simulink model "qss_saab93_ideal"  (R2016b)
settings: Solver=VariableStepDiscrete  StartTime=0.0  StopTime=1220  RelTol=1e-3  EnableMultiTasking=on
undefined symbols (not defined in the file or in its folder): eta_ice, g, h, H_u, k_cs, P_CE_idle, P_CE_recup, rho, rho_f
settings Model: Creator=grauers  LastModifiedBy=grauers
settings DataIOCC: LimitDataPoints=on  SaveFormat=Array  SignalLoggingSaveFormat=ModelDataLogs
settings OptimizationCC: InitFltsAndDblsToZero=on  LifeSpan=inf
settings DebuggingCC: SaveWithParameterizedLinksMsg=none  UnderspecifiedInitializationDetection=Classic  MergeDetectMultiDrivingBlocksExec=none  SignalResolutionControl=TryResolveAllWithWarning  SolverPrmCheckMsg=warning  MultiTaskDSMMsg=warning  MultiTaskCondExecSysMsg=none  FcnCallInpInsideContextMsg=warning  SFUnexpectedBacktrackingDiag=warning  SFNoUnconditionalDefaultTransitionDiag=warning  SFExecutionAtInitializationDiag=none
settings HardwareCC: ProdBitPerPointer=32  ProdBitPerSizeT=32  ProdBitPerPtrDiffT=32  ProdLargestAtomicFloat=None  ProdIntDivRoundTo=Undefined  ProdEndianess=Unspecified  ProdWordSize=32  ProdHWDeviceType=32-bit Generic
settings ModelReferenceCC: PropagateSignalLabelsOutOfModel=off
settings GRTTargetCC: TargetFcnLib=ansi_tfl_tmw.mat  TargetLangStandard=C89/C90 (ANSI)  CombineOutputUpdateFcns=off  GRTInterface=on
settings ConfigComp: CovMetricSettings=dw  CovHtmlReporting=on  CovSaveCumulativeToWorkspaceVar=on  CovSaveSingleToWorkspaceVar=on  CovExternalEMLEnable=off

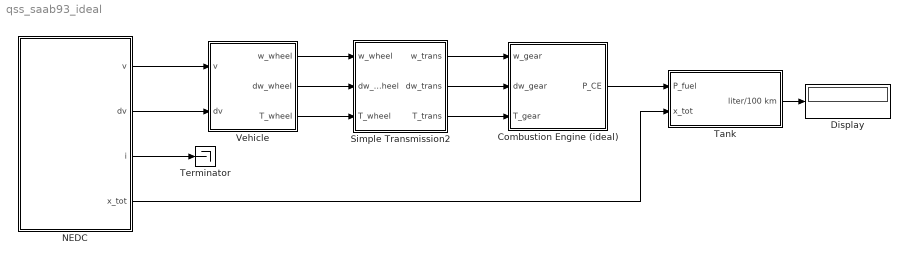
== system qss_saab93_ideal ==
  Combustion Engine (ideal) : Subsystem  Tag=combustion engine  mask(Combustion Engine (ideal)){engine_type=Otto, theta_CE=0.05, P_aux=0, recuperation=No_recuperation, idling=on, idle_power=2600}
      mask prompts: engine_type "Engine type"; theta_CE "Engine inertia [kg*m^2]"; P_aux "Power required by auxiliaries [W]"; recuperation "Recuperation of energy"; idling "Idling power consumption"; idle_power "Idling power consumption [W]"
      mask help:
      | This block simulates the behaviour of a combustion engine. The block is based on an ideal power supply. If engine type ideal is selected then the engine efficiency is 1, else it is 0.4 for otto and 0.5 for diesel.
      |
      | Input:
      | =====
      | 	w_gear		Speed of the fly wheel [rad/s]
      | 	dw_gear	Acceleration of the fly wheel [rad/s^2]
      | 	T_gear		Torque on the fly wheel [Nm]
      |
      | Output:
      | ======
      | 	P_CE		Power produced by the combustion engine [W]
      mask init:
      | init_CE_ideal;
      mask TypeOptions engine_type: Otto | Diesel
      mask TypeOptions recuperation: No_recuperation | Perfect_recuperation
  Display : Display
  NEDC : Subsystem  Tag=cycle  mask(Driving Cycle){cyclename1=NEDC, stepsize=1, autostop=on}
      mask prompts: cyclename1 "Choose a cycle"; stepsize "Step size [s]"; autostop "Enable automatic simulation stop"
      mask help:
      | This block loads the cycle data such as time, speed, acceleration and gear number,  from the specified data file and makes it available on the output of the cycle block.
      |
      | Output:
      | ======
      | 	v	Speed [m/s]
      | 	dv	Acceleration [m/s^2]
      | 	i	Gear number [-]
      | 	x_tot	Total distance [m]
      |
      | Tip:
      | ===
      | Probably you don't need the gear number "i". If so you can terminate
      | it with a "Terminator" out of the "Simulink Library/Connections."
      |
      | Driving cycle:
      | ===
      | Select a driving cycle from the list below or specify your own (place your .mat file in the
      | directory Data/DrivingCycles/UserDefined)
      |
      | ECE_MAN
      | ECE_R15s
      | ECE_R15
      | EUDC
      | EUDC_MAN
      | City
      | City_MAN
      | NEDC
      | NEDC_MANl
      | GOT1
      | GOT2
      | GOT3
      | 10_15_MODE
      | 10_MODE
      | 10_MODE_3
      | 11_MODE
      | 11_MODE_4
      | 15_MODE
      | City_I
      | City_II
      | FTP_75
      | FTP_Highway
      |
      |
      | Step size:
      | ========
      | Default value is 1. Don't change it, unless you are familiar with the programs of the QSS TB.
      |
      | Enable automatic simulation stop:
      | ===========================
      | Stops the simulation automatically at the end of the cycle.
      | Be careful: If you have a component in your model that has to run after the cycle has finished, e.g. a battery to charge, remove the mark!
      mask init:
      | init_driving_cycle1;
      mask Display: plot(T_zplot, V_zplot);
  Simple Transmission2 : Subsystem  Tag=simple transmission  mask(Simple Transmission2){}
      mask help:
      | This block simulates an ideal transmission (no losses).
      |
      | Input:
      | =====
      | 	w_wheel	Speed of the wheel [rad/s]
      | 	dw_wheel	Acceleration of the wheel [rad/s^2]
      | 	T_wheel	Torque on the wheel [Nm]
      |
      | Output:
      | ======
      | 	w_trans		Speed of the fly wheel [rad/s]
      | 	dw_trans	Acceleration of the fly wheel [rad/s^2]
      | 	T_trans		Torque on the fly wheel [Nm]
      mask init:
      | init_transmission;
  Tank : Subsystem  Tag=tank  mask(Tank){fuel=Gasoline, flag_cold_start=off}
      mask prompts: flag_cold_start "Include cold start losses"
      mask help:
      | This block integrates the power (the fuel mass flow) required by the combustion engine or the fuel cell and calculates the energy consumption in liter/100 km.
      |
      | Input:
      | =====
      | 	P_fuel	Power (fuel mass flow) required [W]
      | 	x_tot	Total distance [m]
      |
      | Output:
      | ======
      | 	V	Fuel consumption [liter/100 km]
      mask init:
      | init_tank;
      mask TypeOptions fuel: Gasoline | Diesel | Hydrogen
  Terminator : Terminator
  Vehicle : Subsystem  Tag=vehicle  mask(Vehicle){m_f=1295+80+100, mt2m_f=5, A_f=2, d_wheel=0.62, cw=0.3, mu=0.013}
      mask prompts: m_f "Total mass of the vehicle [kg]"; mt2m_f "Rotating mass [%]"; A_f "Vehicle cross section [m^2]"; d_wheel "Wheel diameter [m]"; cw "Drag coefficient [-]"; mu "Rolling friction coefficient [-]"
      mask help:
      | This block computes the power required from the vehicle.
      |
      | Input:
      | =====
      | 	v		Speed [m/s]
      | 	dv		Acceleration [m/s^2]
      |
      | Output:
      | ======
      | 	w_wheel	Speed of the wheel [rad/s]
      | 	dw_wheel	Acceleration of the wheel [rad/s^2]
      | 	T_wheel	Torque on the wheel [Nm]
      mask init:
      | init_vehicle;
  wires:
  Vehicle/1(w_wheel) -> Simple Transmission2/1(w_wheel)
  Vehicle/2(dw_wheel) -> Simple Transmission2/2(dw_wheel)
  Vehicle/3(T_wheel) -> Simple Transmission2/3(T_wheel)
  Simple Transmission2/1(w_trans) -> Combustion Engine (ideal)/1(w_gear)
  Simple Transmission2/2(dw_trans) -> Combustion Engine (ideal)/2(dw_gear)
  Simple Transmission2/3(T_trans) -> Combustion Engine (ideal)/3(T_gear)
  Tank/1(liter/100 km) -> Display/1
  Combustion Engine (ideal)/1(P_CE) -> Tank/1(P_fuel)
  NEDC/4(x_tot) -> Tank/2(x_tot)
  NEDC/1(v) -> Vehicle/1(v)
  NEDC/2(dv) -> Vehicle/2(dv)
  NEDC/3(i) -> Terminator/1

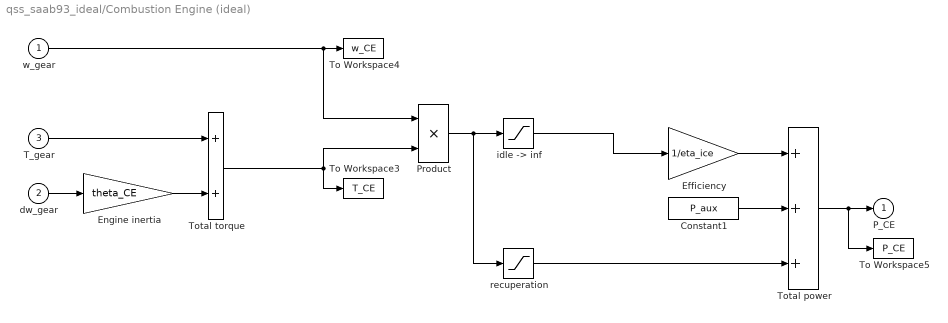
== system qss_saab93_ideal/Combustion Engine (ideal) ==
  w_gear : Inport
  dw_gear : Inport  Port=2
  T_gear : Inport  Port=3
  Constant1 : Constant  Value=P_aux
  Efficiency : Gain  Gain=1/eta_ice  SaturateOnIntegerOverflow=on  OutDataTypeStr=Inherit: Same as input  ParamDataTypeStr=Inherit: Same as input
  Engine inertia : Gain  Gain=theta_CE  SaturateOnIntegerOverflow=on  OutDataTypeStr=Inherit: Same as input  ParamDataTypeStr=Inherit: Same as input
  Product : Product  RndMeth=Zero
  To Workspace3 : ToWorkspace  VariableName=T_CE  SampleTime=-1
  To Workspace4 : ToWorkspace  VariableName=w_CE  SampleTime=-1
  To Workspace5 : ToWorkspace  VariableName=P_CE  SampleTime=-1
  Total power : Sum  Inputs=+++  SaturateOnIntegerOverflow=on  InputSameDT=on  OutDataTypeStr=Inherit: Same as first input
  Total torque : Sum  SaturateOnIntegerOverflow=on  InputSameDT=on  OutDataTypeStr=Inherit: Same as first input
  "idle -> inf" : Saturate  UpperLimit=inf  LowerLimit=P_CE_idle
  recuperation : Saturate  UpperLimit=0  LowerLimit=P_CE_recup
  P_CE : Outport  InitialOutput=0
  wires:
  T_gear/1 -> Total torque/1
  dw_gear/1 -> Engine inertia/1
  Total torque/1 -> Product/2, To Workspace3/1
  Engine inertia/1 -> Total torque/2
  w_gear/1 -> Product/1, To Workspace4/1
  Product/1 -> "idle -> inf"/1, recuperation/1
  Efficiency/1 -> Total power/1
  Total power/1 -> P_CE/1, To Workspace5/1
  Constant1/1 -> Total power/2
  "idle -> inf"/1 -> Efficiency/1
  recuperation/1 -> Total power/3

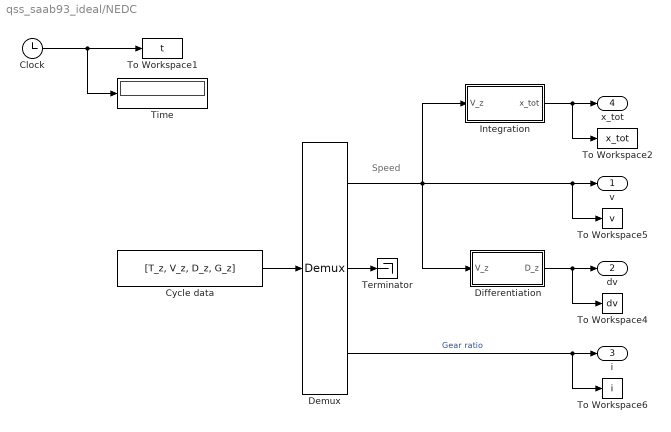
== system qss_saab93_ideal/NEDC ==
  note: Speed
  Clock : Clock
  Cycle data : FromWorkspace  VariableName=[T_z, V_z, D_z, G_z]  SampleTime=h
  Demux : Demux  Outputs=3
  Differentiation : Subsystem
  Integration : Subsystem
  Terminator : Terminator
  Time : Display
  To Workspace1 : ToWorkspace  VariableName=t  SampleTime=-1
  To Workspace2 : ToWorkspace  VariableName=x_tot  SampleTime=-1
  To Workspace4 : ToWorkspace  VariableName=dv  SampleTime=-1
  To Workspace5 : ToWorkspace  VariableName=v  SampleTime=-1
  To Workspace6 : ToWorkspace  VariableName=i  SampleTime=-1
  v : Outport  InitialOutput=0
  dv : Outport  Port=2  InitialOutput=0
  i : Outport  Port=3  InitialOutput=0
  x_tot : Outport  Port=4  InitialOutput=0
  wires:
  Clock/1 -> To Workspace1/1, Time/1
  Demux/3 -> To Workspace6/1, i/1  "Gear ratio"
  Integration/1(x_tot) -> To Workspace2/1, x_tot/1
  Demux/1 -> Differentiation/1(V_z), To Workspace5/1, v/1, Integration/1(V_z)
  Demux/2 -> Terminator/1
  Differentiation/1(D_z) -> dv/1, To Workspace4/1
  Cycle data/1 -> Demux/1

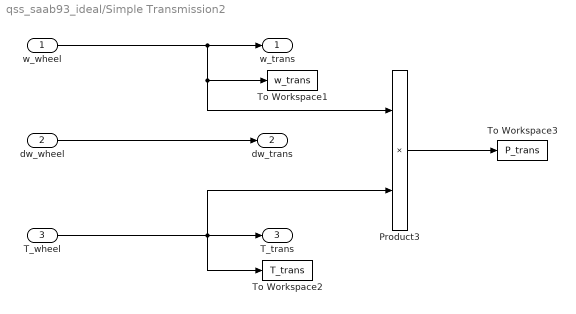
== system qss_saab93_ideal/Simple Transmission2 ==
  w_wheel : Inport
  dw_wheel : Inport  Port=2
  T_wheel : Inport  Port=3
  Product3 : Product  SaturateOnIntegerOverflow=on  RndMeth=Zero  InputSameDT=on  OutDataTypeStr=Inherit: Same as first input
  To Workspace1 : ToWorkspace  VariableName=w_trans  SampleTime=-1
  To Workspace2 : ToWorkspace  VariableName=T_trans  SampleTime=-1
  To Workspace3 : ToWorkspace  VariableName=P_trans  SampleTime=-1
  w_trans : Outport  InitialOutput=0
  dw_trans : Outport  Port=2  InitialOutput=0
  T_trans : Outport  Port=3  InitialOutput=0
  wires:
  Product3/1 -> To Workspace3/1
  w_wheel/1 -> w_trans/1, Product3/1, To Workspace1/1
  T_wheel/1 -> Product3/2, T_trans/1, To Workspace2/1
  dw_wheel/1 -> dw_trans/1

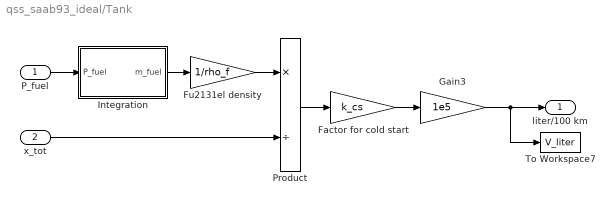
== system qss_saab93_ideal/Tank ==
  P_fuel : Inport
  x_tot : Inport  Port=2
  Factor for cold start : Gain  Gain=k_cs  SaturateOnIntegerOverflow=on  OutDataTypeStr=Inherit: Same as input  ParamDataTypeStr=Inherit: Same as input
  Fu2131el density : Gain  Gain=1/rho_f  SaturateOnIntegerOverflow=on  OutDataTypeStr=Inherit: Same as input  ParamDataTypeStr=Inherit: Same as input
  Gain3 : Gain  Gain=1e5  SaturateOnIntegerOverflow=on  OutDataTypeStr=Inherit: Same as input  ParamDataTypeStr=Inherit: Same as input
  Integration : Subsystem
  Product : Product  Inputs=*/  SaturateOnIntegerOverflow=on  RndMeth=Zero  InputSameDT=on  OutDataTypeStr=Inherit: Same as first input
  To Workspace7 : ToWorkspace  VariableName=V_liter  SampleTime=-1
  liter/100 km : Outport  InitialOutput=0
  wires:
  Factor for cold start/1 -> Gain3/1
  Product/1 -> Factor for cold start/1
  Fu2131el density/1 -> Product/1
  Gain3/1 -> To Workspace7/1, liter/100 km/1
  Integration/1(m_fuel) -> Fu2131el density/1
  x_tot/1 -> Product/2
  P_fuel/1 -> Integration/1(P_fuel)

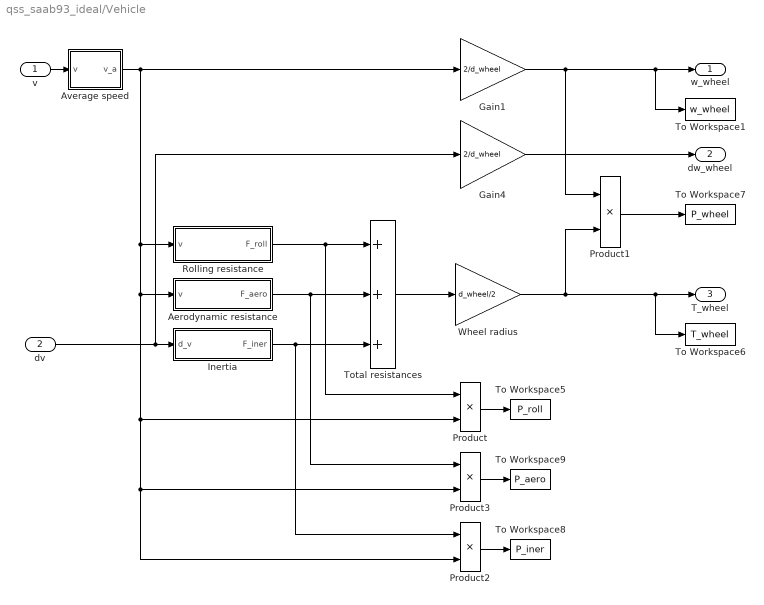
== system qss_saab93_ideal/Vehicle ==
  v : Inport
  dv : Inport  Port=2
  Aerodynamic resistance : Subsystem
  Average speed : Subsystem
  Gain1 : Gain  Gain=2/d_wheel  SaturateOnIntegerOverflow=on  OutDataTypeStr=Inherit: Same as input  ParamDataTypeStr=Inherit: Same as input
  Gain4 : Gain  Gain=2/d_wheel  SaturateOnIntegerOverflow=on  OutDataTypeStr=Inherit: Same as input  ParamDataTypeStr=Inherit: Same as input
  Inertia : Subsystem
  Product{,1..3} (4 alike) : Product  SaturateOnIntegerOverflow=on  RndMeth=Zero  InputSameDT=on  OutDataTypeStr=Inherit: Same as first input
  Rolling resistance : Subsystem
  To Workspace1 : ToWorkspace  VariableName=w_wheel  SampleTime=-1
  To Workspace5 : ToWorkspace  VariableName=P_roll  SampleTime=-1
  To Workspace6 : ToWorkspace  VariableName=T_wheel  SampleTime=-1
  To Workspace7 : ToWorkspace  VariableName=P_wheel  SampleTime=-1
  To Workspace8 : ToWorkspace  VariableName=P_iner  SampleTime=-1
  To Workspace9 : ToWorkspace  VariableName=P_aero  SampleTime=-1
  Total resistances : Sum  Inputs=+++  SaturateOnIntegerOverflow=on  InputSameDT=on  OutDataTypeStr=Inherit: Same as first input
  Wheel radius : Gain  Gain=d_wheel/2  SaturateOnIntegerOverflow=on  OutDataTypeStr=Inherit: Same as input  ParamDataTypeStr=Inherit: Same as input
  w_wheel : Outport  InitialOutput=0
  dw_wheel : Outport  Port=2  InitialOutput=0
  T_wheel : Outport  Port=3  InitialOutput=0
  wires:
  Product/1 -> To Workspace5/1
  Product1/1 -> To Workspace7/1
  Product3/1 -> To Workspace9/1
  Product2/1 -> To Workspace8/1
  v/1 -> Average speed/1(v)
  dv/1 -> Gain4/1, Inertia/1(d_v)
  Average speed/1(v_a) -> Rolling resistance/1(v), Product2/2, Product3/2, Product/2, Aerodynamic resistance/1(v), Gain1/1
  Wheel radius/1 -> To Workspace6/1, T_wheel/1, Product1/2
  Total resistances/1 -> Wheel radius/1
  Inertia/1(F_iner) -> Product2/1, Total resistances/3
  Aerodynamic resistance/1(F_aero) -> Total resistances/2, Product3/1
  Rolling resistance/1(F_roll) -> Product/1, Total resistances/1
  Gain1/1 -> To Workspace1/1, w_wheel/1, Product1/1
  Gain4/1 -> dw_wheel/1

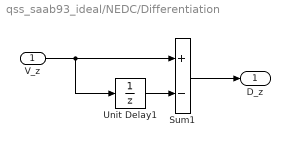
== system qss_saab93_ideal/NEDC/Differentiation ==
  V_z : Inport
  Sum1 : Sum  Inputs=+-  SaturateOnIntegerOverflow=on  InputSameDT=on  OutDataTypeStr=Inherit: Same as first input
  Unit Delay1 : UnitDelay  SampleTime=h
  D_z : Outport  InitialOutput=0
  wires:
  Sum1/1 -> D_z/1
  V_z/1 -> Unit Delay1/1, Sum1/1
  Unit Delay1/1 -> Sum1/2

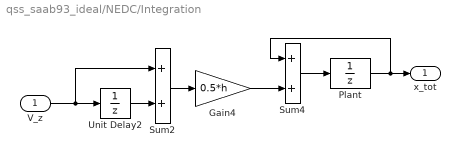
== system qss_saab93_ideal/NEDC/Integration ==
  V_z : Inport
  Gain4 : Gain  Gain=0.5*h  SaturateOnIntegerOverflow=on  OutDataTypeStr=Inherit: Same as input  ParamDataTypeStr=Inherit: Same as input
  Plant : UnitDelay  InitialCondition=1  SampleTime=h
  Sum2 : Sum  SaturateOnIntegerOverflow=on  InputSameDT=on  OutDataTypeStr=Inherit: Same as first input
  Sum4 : Sum  SaturateOnIntegerOverflow=on  InputSameDT=on  OutDataTypeStr=Inherit: Same as first input
  Unit Delay2 : UnitDelay  SampleTime=h
  x_tot : Outport  InitialOutput=0
  wires:
  Plant/1 -> x_tot/1, Sum4/1
  Sum4/1 -> Plant/1
  Gain4/1 -> Sum4/2
  V_z/1 -> Unit Delay2/1, Sum2/1
  Unit Delay2/1 -> Sum2/2
  Sum2/1 -> Gain4/1

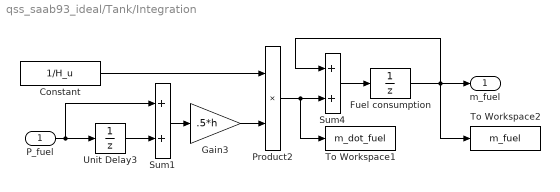
== system qss_saab93_ideal/Tank/Integration ==
  P_fuel : Inport
  Constant : Constant  Value=1/H_u
  Fuel consumption : UnitDelay  SampleTime=h
  Gain3 : Gain  Gain=.5*h  SaturateOnIntegerOverflow=on  OutDataTypeStr=Inherit: Same as input  ParamDataTypeStr=Inherit: Same as input
  Product2 : Product  SaturateOnIntegerOverflow=on  RndMeth=Zero  InputSameDT=on  OutDataTypeStr=Inherit: Same as first input
  Sum1 : Sum  SaturateOnIntegerOverflow=on  InputSameDT=on  OutDataTypeStr=Inherit: Same as first input
  Sum4 : Sum  SaturateOnIntegerOverflow=on  InputSameDT=on  OutDataTypeStr=Inherit: Same as first input
  To Workspace1 : ToWorkspace  VariableName=m_dot_fuel  SampleTime=-1
  To Workspace2 : ToWorkspace  VariableName=m_fuel  SampleTime=-1
  Unit Delay3 : UnitDelay  SampleTime=h
  m_fuel : Outport  InitialOutput=0
  wires:
  Product2/1 -> To Workspace1/1, Sum4/2
  Sum4/1 -> Fuel consumption/1
  Fuel consumption/1 -> To Workspace2/1, Sum4/1, m_fuel/1
  Sum1/1 -> Gain3/1
  Unit Delay3/1 -> Sum1/2
  P_fuel/1 -> Unit Delay3/1, Sum1/1
  Gain3/1 -> Product2/2
  Constant/1 -> Product2/1

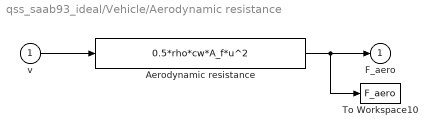
== system qss_saab93_ideal/Vehicle/Aerodynamic resistance ==
  v : Inport
  Aerodynamic resistance : Fcn  Expr=0.5*rho*cw*A_f*u^2
  To Workspace10 : ToWorkspace  VariableName=F_aero  SampleTime=-1
  F_aero : Outport  InitialOutput=0
  wires:
  Aerodynamic resistance/1 -> To Workspace10/1, F_aero/1
  v/1 -> Aerodynamic resistance/1

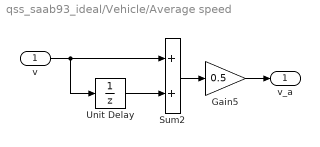
== system qss_saab93_ideal/Vehicle/Average speed ==
  v : Inport
  Gain5 : Gain  Gain=0.5  SaturateOnIntegerOverflow=on  OutDataTypeStr=Inherit: Same as input  ParamDataTypeStr=Inherit: Same as input
  Sum2 : Sum  SaturateOnIntegerOverflow=on  InputSameDT=on  OutDataTypeStr=Inherit: Same as first input
  Unit Delay : UnitDelay  SampleTime=h
  v_a : Outport  InitialOutput=0
  wires:
  v/1 -> Unit Delay/1, Sum2/1
  Gain5/1 -> v_a/1
  Sum2/1 -> Gain5/1
  Unit Delay/1 -> Sum2/2

== system qss_saab93_ideal/Vehicle/Inertia ==
  d_v : Inport
  Inertia : Fcn  Expr=m_f*(1+mt2m_f/100)*u/h
  To Workspace10 : ToWorkspace  VariableName=F_iner  SampleTime=-1
  F_iner : Outport  InitialOutput=0
  wires:
  d_v/1 -> Inertia/1
  Inertia/1 -> To Workspace10/1, F_iner/1

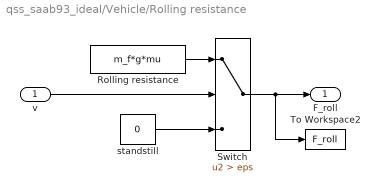
== system qss_saab93_ideal/Vehicle/Rolling resistance ==
  v : Inport
  Rolling resistance : Constant  Value=m_f*g*mu
  Switch : Switch  Criteria=u2 > Threshold  Threshold=eps
  To Workspace2 : ToWorkspace  VariableName=F_roll  SampleTime=-1
  standstill : Constant  Value=0
  F_roll : Outport
  wires:
  Rolling resistance/1 -> Switch/1
  standstill/1 -> Switch/3
  v/1 -> Switch/2
  Switch/1 -> F_roll/1, To Workspace2/1
